simulink model "model_lineaire"  (R2021b)
settings: Solver=VariableStepAuto  StartTime=0.0  StopTime=10.0  RelTol=1e-3
values from neighbouring files (symbols this model uses):
  Ax_e = 0    [equation_lineaire.m]
  Ay_e = 0    [equation_lineaire.m]
  Ia_e = 0    [equation_lineaire.m]
  Ib_e = 0    [equation_lineaire.m]
  Ic_e = 0    [equation_lineaire.m]
  Px_e = 0    [equation_lineaire.m]
  Py_e = 0    [equation_lineaire.m]
  Pz_e = 0    [equation_lineaire.m]
  Vx_e = 0    [equation_lineaire.m]
  Vy_e = 0    [equation_lineaire.m]
  Wx_e = 0    [equation_lineaire.m]
  Wy_e = 0    [equation_lineaire.m]
undefined symbols (not defined in the file or in its folder): A_lineaire, B_lineaire, C_lineaire, C_variable_etat, D_lineaire, D_variable_etat, Va_e, Vb_e, Vc_e, Vz_e, zD_e, zE_e, zF_e
settings Model: Creator=alexi  LastModifiedBy=alexi

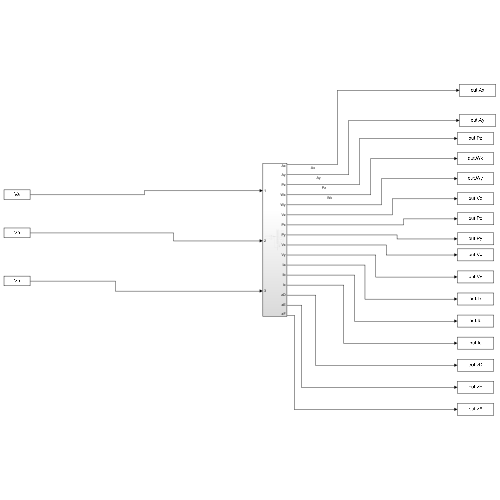
[thumbnail: Simulink's stored preview of the top-level diagram]
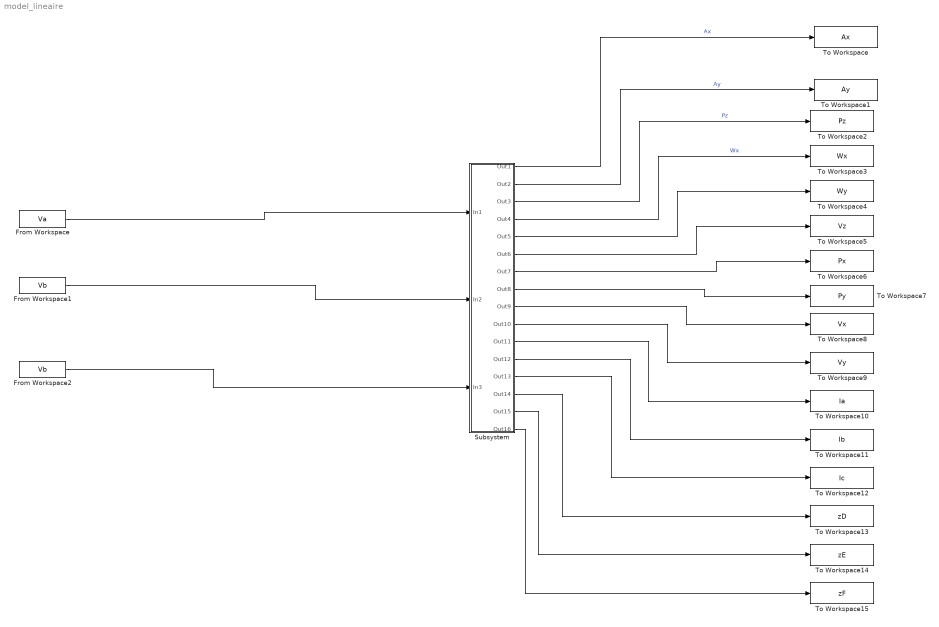
== system model_lineaire ==
  From Workspace : FromWorkspace  VariableName=Va
  From Workspace1 : FromWorkspace  VariableName=Vb
  From Workspace2 : FromWorkspace  VariableName=Vb
  Subsystem : Subsystem
  To Workspace : ToWorkspace  VariableName=Ax  SaveFormat=Timeseries  SampleTime=-1
  To Workspace1 : ToWorkspace  VariableName=Ay  SaveFormat=Timeseries  SampleTime=-1
  To Workspace10 : ToWorkspace  VariableName=Ia  SaveFormat=Timeseries  SampleTime=-1
  To Workspace11 : ToWorkspace  VariableName=Ib  SaveFormat=Timeseries  SampleTime=-1
  To Workspace12 : ToWorkspace  VariableName=Ic  SaveFormat=Timeseries  SampleTime=-1
  To Workspace13 : ToWorkspace  VariableName=zD  SaveFormat=Timeseries  SampleTime=-1
  To Workspace14 : ToWorkspace  VariableName=zE  SaveFormat=Timeseries  SampleTime=-1
  To Workspace15 : ToWorkspace  VariableName=zF  SaveFormat=Timeseries  SampleTime=-1
  To Workspace2 : ToWorkspace  VariableName=Pz  SaveFormat=Timeseries  SampleTime=-1
  To Workspace3 : ToWorkspace  VariableName=Wx  SaveFormat=Timeseries  SampleTime=-1
  To Workspace4 : ToWorkspace  VariableName=Wy  SaveFormat=Timeseries  SampleTime=-1
  To Workspace5 : ToWorkspace  VariableName=Vz  SaveFormat=Timeseries  SampleTime=-1
  To Workspace6 : ToWorkspace  VariableName=Px  SaveFormat=Timeseries  SampleTime=-1
  To Workspace7 : ToWorkspace  VariableName=Py  SaveFormat=Timeseries  SampleTime=-1
  To Workspace8 : ToWorkspace  VariableName=Vx  SaveFormat=Timeseries  SampleTime=-1
  To Workspace9 : ToWorkspace  VariableName=Vy  SaveFormat=Timeseries  SampleTime=-1
  wires:
  From Workspace/1 -> Subsystem/1(In1)
  From Workspace1/1 -> Subsystem/2(In2)
  From Workspace2/1 -> Subsystem/3(In3)
  Subsystem/1(Out1) -> To Workspace/1  "Ax"
  Subsystem/2(Out2) -> To Workspace1/1  "Ay"
  Subsystem/3(Out3) -> To Workspace2/1  "Pz"
  Subsystem/4(Out4) -> To Workspace3/1  "Wx"
  Subsystem/5(Out5) -> To Workspace4/1
  Subsystem/6(Out6) -> To Workspace5/1
  Subsystem/7(Out7) -> To Workspace6/1
  Subsystem/8(Out8) -> To Workspace7/1
  Subsystem/9(Out9) -> To Workspace8/1
  Subsystem/10(Out10) -> To Workspace9/1
  Subsystem/11(Out11) -> To Workspace10/1
  Subsystem/12(Out12) -> To Workspace11/1
  Subsystem/13(Out13) -> To Workspace12/1
  Subsystem/14(Out14) -> To Workspace13/1
  Subsystem/15(Out15) -> To Workspace14/1
  Subsystem/16(Out16) -> To Workspace15/1

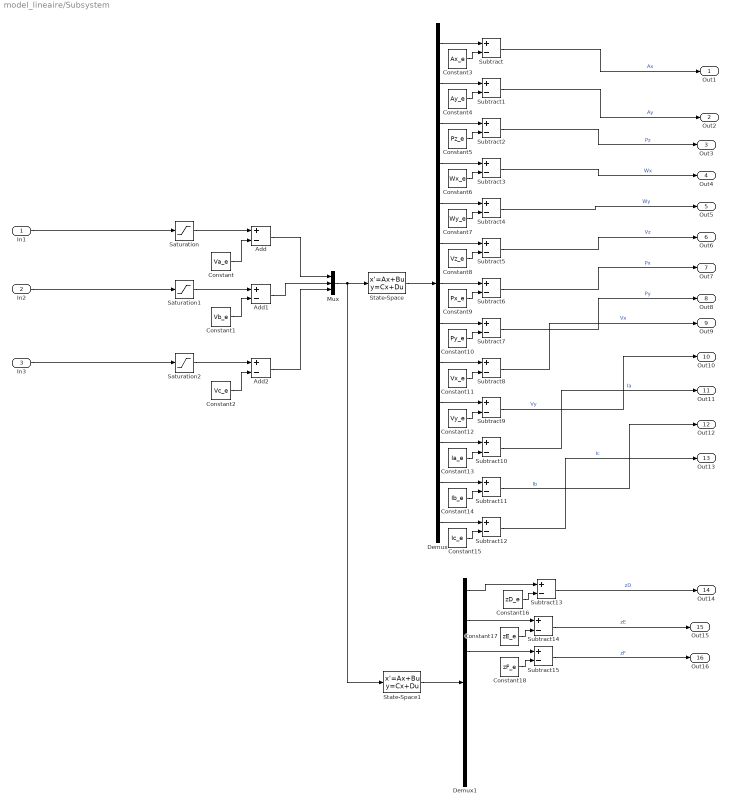
== system model_lineaire/Subsystem ==
  In1 : Inport
  In2 : Inport  Port=2
  In3 : Inport  Port=3
  Add : Sum  Inputs=+-
  Add1 : Sum  Inputs=+-
  Add2 : Sum  Inputs=+-
  Constant : Constant  Value=Va_e
  Constant1 : Constant  Value=Vb_e
  Constant10 : Constant  Value=Py_e
  Constant11 : Constant  Value=Vx_e
  Constant12 : Constant  Value=Vy_e
  Constant13 : Constant  Value=Ia_e
  Constant14 : Constant  Value=Ib_e
  Constant15 : Constant  Value=Ic_e
  Constant16 : Constant  Value=zD_e
  Constant17 : Constant  Value=zE_e
  Constant18 : Constant  Value=zF_e
  Constant2 : Constant  Value=Vc_e
  Constant3 : Constant  Value=Ax_e
  Constant4 : Constant  Value=Ay_e
  Constant5 : Constant  Value=Pz_e
  Constant6 : Constant  Value=Wx_e
  Constant7 : Constant  Value=Wy_e
  Constant8 : Constant  Value=Vz_e
  Constant9 : Constant  Value=Px_e
  Demux : Demux  Outputs=13
  Demux1 : Demux  Outputs=7
  Mux : Mux  Inputs=3
  Saturation : Saturate
  Saturation1 : Saturate
  Saturation2 : Saturate
  State-Space : StateSpace  A=A_lineaire  B=B_lineaire  C=C_variable_etat  D=D_variable_etat  InitialCondition=0
  State-Space1 : StateSpace  A=A_lineaire  B=B_lineaire  C=C_lineaire  D=D_lineaire  InitialCondition=0
  Subtract{,1..15} (16 alike) : Sum  Inputs=+-
  Out1 : Outport
  Out2 : Outport  Port=2
  Out3 : Outport  Port=3
  Out4 : Outport  Port=4
  Out5 : Outport  Port=5
  Out6 : Outport  Port=6
  Out7 : Outport  Port=7
  Out8 : Outport  Port=8
  Out9 : Outport  Port=9
  Out10 : Outport  Port=10
  Out11 : Outport  Port=11
  Out12 : Outport  Port=12
  Out13 : Outport  Port=13
  Out14 : Outport  Port=14
  Out15 : Outport  Port=15
  Out16 : Outport  Port=16
  wires:
  Constant7/1 -> Subtract4/2
  Saturation2/1 -> Add2/1
  Demux/7 -> Subtract6/1
  Subtract/1 -> Out1/1  "Ax"
  State-Space/1 -> Demux/1
  Subtract8/1 -> Out9/1  "Vx"
  Subtract10/1 -> Out11/1  "Ia"
  Demux/5 -> Subtract4/1
  Subtract4/1 -> Out5/1  "Wy"
  Constant4/1 -> Subtract1/2
  Subtract2/1 -> Out3/1  "Pz"
  Constant15/1 -> Subtract12/2
  Demux/3 -> Subtract2/1
  Demux/8 -> Subtract7/1
  Constant11/1 -> Subtract8/2
  Constant2/1 -> Add2/2
  Constant13/1 -> Subtract10/2
  Constant5/1 -> Subtract2/2
  In2/1 -> Saturation1/1
  Demux/11 -> Subtract10/1
  Demux/6 -> Subtract5/1
  Demux/4 -> Subtract3/1
  Constant8/1 -> Subtract5/2
  Demux/9 -> Subtract8/1
  Saturation/1 -> Add/1
  Constant/1 -> Add/2
  Add2/1 -> Mux/3
  Subtract12/1 -> Out13/1  "Ic"
  Mux/1 -> State-Space1/1, State-Space/1
  Demux/1 -> Subtract/1
  Subtract11/1 -> Out12/1  "Ib"
  Constant1/1 -> Add1/2
  Demux/2 -> Subtract1/1
  Add1/1 -> Mux/2
  Demux/12 -> Subtract11/1
  Constant3/1 -> Subtract/2
  Constant10/1 -> Subtract7/2
  Constant12/1 -> Subtract9/2
  Subtract5/1 -> Out6/1  "Vz"
  Demux/10 -> Subtract9/1
  Constant6/1 -> Subtract3/2
  Demux/13 -> Subtract12/1
  Subtract9/1 -> Out10/1  "Vy"
  Constant9/1 -> Subtract6/2
  Saturation1/1 -> Add1/1
  Constant14/1 -> Subtract11/2
  Add/1 -> Mux/1
  In3/1 -> Saturation2/1
  Subtract7/1 -> Out8/1  "Py"
  Subtract3/1 -> Out4/1  "Wx"
  Subtract1/1 -> Out2/1  "Ay"
  Subtract6/1 -> Out7/1  "Px"
  In1/1 -> Saturation/1
  State-Space1/1 -> Demux1/1
  Demux1/1 -> Subtract13/1
  Constant16/1 -> Subtract13/2
  Constant17/1 -> Subtract14/2
  Demux1/2 -> Subtract14/1
  Demux1/3 -> Subtract15/1
  Constant18/1 -> Subtract15/2
  Subtract13/1 -> Out14/1  "zD"
  Subtract14/1 -> Out15/1  "zE"
  Subtract15/1 -> Out16/1  "zF"
